simulink model "bh_4dof_LAGR_manipulator_CONTROL_DL_discrete"  (R2016b)
settings: Solver=ode15s  StartTime=0.0  StopTime=60  FixedStep=0.001  RelTol=1e-5  EnableMultiTasking=on
undefined symbols (not defined in the file or in its folder): b1_damp, b2_damp, b3_damp, b4_damp, g, Hz, L1x, L1y, L1z, L2x, L2y, L2z, L3x, L3y, L3z, mass1, mass2, mass3, mass4, Rturn, theta1_0, theta1_dot_0, theta2_0, theta2_dot_0, theta3_0, theta3_dot_0, theta4_0, theta4_dot_0, X, Y, Z
libraries: sm_lib x25, nesl_utility x17, simulink x9, discretizing x4, simulink_extras x2
(part 2 of 3)

== system bh_4dof_LAGR_manipulator_CONTROL_DL_discrete/CONTROL_LAW/CLAW_LINK2 ==
  note: Rise Settle
      | VEL LOOP 0.0056 0.01
      | POS LOOP 0.0274 0.05
  FFWD : Inport
  CMD_POS : Inport  Port=2
  MEAS_POS : Inport  Port=3
  MEAS_VEL : Inport  Port=4
  Constant : Constant
  Manual Switch : ManualSwitch  CurrentSetting=0
  PID Controller : simulink/Continuous/PID Controller  Controller=P  TimeDomain=Discrete-time  SampleTime=0.001  IntegratorMethod=Forward Euler  FilterMethod=Forward Euler  Form=Parallel  UseFilter=on  ControllerParametersSource=internal  P=64.6199485469639  I=1  D=0  N=100  InitialConditionSource=internal  InitialConditionForIntegrator=0  InitialConditionForFilter=0  ExternalReset=none  LimitOutput=off  UpperSaturationLimit=inf  LowerSaturationLimit=-inf  LinearizeAsGain=on  AntiWindupMode=none  Kb=1  TrackingMode=off  Kt=1  PParamMin=[]  PParamMax=[]  IParamMin=[]  IParamMax=[]  DParamMin=[]  DParamMax=[]  NParamMin=[]  NParamMax=[]  KbParamMin=[]  KbParamMax=[]  KtParamMin=[]  KtParamMax=[]  POutMin=[]  POutMax=[]  IOutMin=[]  IOutMax=[]  DOutMin=[]  DOutMax=[]  NOutMin=[]  NOutMax=[]  KbOutMin=[]  KbOutMax=[]  KtOutMin=[]  KtOutMax=[]  IntegratorOutMin=[]  IntegratorOutMax=[]  FilterOutMin=[]  FilterOutMax=[]  SumOutMin=[]  SumOutMax=[]  SumI1OutMin=[]  SumI1OutMax=[]  SumI2OutMin=[]  SumI2OutMax=[]  SumI3OutMin=[]  SumI3OutMax=[]  SumDOutMin=[]  SumDOutMax=[]  SaturationOutMin=[]  SaturationOutMax=[]  IntegratorContinuousStateAttributes=''  IntegratorStateMustResolveToSignalObject=off  IntegratorRTWStateStorageClass=Auto  FilterContinuousStateAttributes=''  FilterStateMustResolveToSignalObject=off  FilterRTWStateStorageClass=Auto  DifferentiatorICPrevScaledInput=0  DifferentiatorOutMin=[]  DifferentiatorOutMax=[]
      settings: AttributesFormatString=DT= %<SampleTime>
  PID Controller1 : simulink/Continuous/PID Controller  Controller=P  TimeDomain=Discrete-time  SampleTime=0.001  IntegratorMethod=Forward Euler  FilterMethod=Forward Euler  Form=Parallel  UseFilter=on  ControllerParametersSource=internal  P=12.0646813225273  I=10  D=0  N=100  InitialConditionSource=internal  InitialConditionForIntegrator=0  InitialConditionForFilter=0  ExternalReset=none  LimitOutput=off  UpperSaturationLimit=inf  LowerSaturationLimit=-inf  LinearizeAsGain=on  AntiWindupMode=none  Kb=1  TrackingMode=off  Kt=1  PParamMin=[]  PParamMax=[]  IParamMin=[]  IParamMax=[]  DParamMin=[]  DParamMax=[]  NParamMin=[]  NParamMax=[]  KbParamMin=[]  KbParamMax=[]  KtParamMin=[]  KtParamMax=[]  POutMin=[]  POutMax=[]  IOutMin=[]  IOutMax=[]  DOutMin=[]  DOutMax=[]  NOutMin=[]  NOutMax=[]  KbOutMin=[]  KbOutMax=[]  KtOutMin=[]  KtOutMax=[]  IntegratorOutMin=[]  IntegratorOutMax=[]  FilterOutMin=[]  FilterOutMax=[]  SumOutMin=[]  SumOutMax=[]  SumI1OutMin=[]  SumI1OutMax=[]  SumI2OutMin=[]  SumI2OutMax=[]  SumI3OutMin=[]  SumI3OutMax=[]  SumDOutMin=[]  SumDOutMax=[]  SaturationOutMin=[]  SaturationOutMax=[]  IntegratorContinuousStateAttributes=''  IntegratorStateMustResolveToSignalObject=off  IntegratorRTWStateStorageClass=Auto  FilterContinuousStateAttributes=''  FilterStateMustResolveToSignalObject=off  FilterRTWStateStorageClass=Auto  DifferentiatorICPrevScaledInput=0  DifferentiatorOutMin=[]  DifferentiatorOutMax=[]
      settings: AttributesFormatString=DT= %<SampleTime>
  Sum : Sum  Inputs=|+-
  Sum1 : Sum  Inputs=++|
  Sum2 : Sum  Inputs=+|-
  Transfer Fcn1 : discretizing/Discretized Transfer Fcn  Numerator=[100]  Denominator=[1 100]  AbsTol=auto  SampleTime=0.001  method=tustin  Wc=1
  Transfer Fcn4 : discretizing/Discretized Transfer Fcn  Commented=on  Numerator=[300]  Denominator=[1 300]  AbsTol=auto  SampleTime=0.001  method=tustin  Wc=1
  TQ : Outport
  wires:
  FFWD/1 -> Sum1/1
  Sum1/1 -> [T], TQ/1
  CMD_POS/1 -> Sum/1
  MEAS_VEL/1 -> Transfer Fcn1/1  "VEL"
  MEAS_POS/1 -> Sum/2  "POS"
  PID Controller/1 -> Manual Switch/2
  Sum2/1 -> PID Controller1/1
  Manual Switch/1 -> Sum2/1, [VZ]
  Constant/1 -> Manual Switch/1
  PID Controller1/1 -> Sum1/2
  Sum/1 -> PID Controller/1
  Transfer Fcn1/1 -> Sum2/2

== system bh_4dof_LAGR_manipulator_CONTROL_DL_discrete/CONTROL_LAW/CLAW_LINK3 ==
  note: Rise Settle
      | VEL LOOP 0.0056 0.01
      | POS LOOP 0.0274 0.05
  FFWD : Inport
  CMD_POS : Inport  Port=2
  MEAS_POS : Inport  Port=3
  MEAS_VEL : Inport  Port=4
  Constant : Constant
  Manual Switch : ManualSwitch  CurrentSetting=0
  PID Controller : simulink/Continuous/PID Controller  Controller=P  TimeDomain=Discrete-time  SampleTime=0.001  IntegratorMethod=Forward Euler  FilterMethod=Forward Euler  Form=Parallel  UseFilter=on  ControllerParametersSource=internal  P=15*4  I=1  D=0  N=100  InitialConditionSource=internal  InitialConditionForIntegrator=0  InitialConditionForFilter=0  ExternalReset=none  LimitOutput=off  UpperSaturationLimit=inf  LowerSaturationLimit=-inf  LinearizeAsGain=on  AntiWindupMode=none  Kb=1  TrackingMode=off  Kt=1  PParamMin=[]  PParamMax=[]  IParamMin=[]  IParamMax=[]  DParamMin=[]  DParamMax=[]  NParamMin=[]  NParamMax=[]  KbParamMin=[]  KbParamMax=[]  KtParamMin=[]  KtParamMax=[]  POutMin=[]  POutMax=[]  IOutMin=[]  IOutMax=[]  DOutMin=[]  DOutMax=[]  NOutMin=[]  NOutMax=[]  KbOutMin=[]  KbOutMax=[]  KtOutMin=[]  KtOutMax=[]  IntegratorOutMin=[]  IntegratorOutMax=[]  FilterOutMin=[]  FilterOutMax=[]  SumOutMin=[]  SumOutMax=[]  SumI1OutMin=[]  SumI1OutMax=[]  SumI2OutMin=[]  SumI2OutMax=[]  SumI3OutMin=[]  SumI3OutMax=[]  SumDOutMin=[]  SumDOutMax=[]  SaturationOutMin=[]  SaturationOutMax=[]  IntegratorContinuousStateAttributes=''  IntegratorStateMustResolveToSignalObject=off  IntegratorRTWStateStorageClass=Auto  FilterContinuousStateAttributes=''  FilterStateMustResolveToSignalObject=off  FilterRTWStateStorageClass=Auto  DifferentiatorICPrevScaledInput=0  DifferentiatorOutMin=[]  DifferentiatorOutMax=[]
      settings: AttributesFormatString=DT= %<SampleTime>
  PID Controller1 : simulink/Continuous/PID Controller  Controller=P  TimeDomain=Discrete-time  SampleTime=0.001  IntegratorMethod=Forward Euler  FilterMethod=Forward Euler  Form=Parallel  UseFilter=on  ControllerParametersSource=internal  P=0.422912648203834  I=10  D=0  N=100  InitialConditionSource=internal  InitialConditionForIntegrator=0  InitialConditionForFilter=0  ExternalReset=none  LimitOutput=off  UpperSaturationLimit=inf  LowerSaturationLimit=-inf  LinearizeAsGain=on  AntiWindupMode=none  Kb=1  TrackingMode=off  Kt=1  PParamMin=[]  PParamMax=[]  IParamMin=[]  IParamMax=[]  DParamMin=[]  DParamMax=[]  NParamMin=[]  NParamMax=[]  KbParamMin=[]  KbParamMax=[]  KtParamMin=[]  KtParamMax=[]  POutMin=[]  POutMax=[]  IOutMin=[]  IOutMax=[]  DOutMin=[]  DOutMax=[]  NOutMin=[]  NOutMax=[]  KbOutMin=[]  KbOutMax=[]  KtOutMin=[]  KtOutMax=[]  IntegratorOutMin=[]  IntegratorOutMax=[]  FilterOutMin=[]  FilterOutMax=[]  SumOutMin=[]  SumOutMax=[]  SumI1OutMin=[]  SumI1OutMax=[]  SumI2OutMin=[]  SumI2OutMax=[]  SumI3OutMin=[]  SumI3OutMax=[]  SumDOutMin=[]  SumDOutMax=[]  SaturationOutMin=[]  SaturationOutMax=[]  IntegratorContinuousStateAttributes=''  IntegratorStateMustResolveToSignalObject=off  IntegratorRTWStateStorageClass=Auto  FilterContinuousStateAttributes=''  FilterStateMustResolveToSignalObject=off  FilterRTWStateStorageClass=Auto  DifferentiatorICPrevScaledInput=0  DifferentiatorOutMin=[]  DifferentiatorOutMax=[]
      settings: AttributesFormatString=DT= %<SampleTime>
  Sum : Sum  Inputs=|+-
  Sum1 : Sum  Inputs=++|
  Sum2 : Sum  Inputs=+|-
  TQ : Outport
  wires:
  FFWD/1 -> Sum1/1
  Sum1/1 -> [T], TQ/1
  CMD_POS/1 -> Sum/1
  MEAS_VEL/1 -> Sum2/2  "VEL"
  MEAS_POS/1 -> Sum/2  "POS"
  Sum2/1 -> PID Controller1/1
  Manual Switch/1 -> Sum2/1, [VZ]
  Constant/1 -> Manual Switch/1
  Sum/1 -> PID Controller/1
  PID Controller1/1 -> Sum1/2
  PID Controller/1 -> Manual Switch/2

== system bh_4dof_LAGR_manipulator_CONTROL_DL_discrete/CONTROL_LAW/CLAW_TURN ==
  note: Settle
      | VEL LOOP 0.01
      | POS LOOP 0.05
  FFWD : Inport
  CMD_POS : Inport  Port=2
  MEAS_POS : Inport  Port=3
  MEAS_VEL : Inport  Port=4
  Constant : Constant
  Manual Switch : ManualSwitch  CurrentSetting=0
  PID Controller : simulink/Continuous/PID Controller  Controller=P  TimeDomain=Discrete-time  SampleTime=0.001  IntegratorMethod=Forward Euler  FilterMethod=Forward Euler  Form=Parallel  UseFilter=on  ControllerParametersSource=internal  P=63.9206057044755  I=1  D=0  N=100  InitialConditionSource=internal  InitialConditionForIntegrator=0  InitialConditionForFilter=0  ExternalReset=none  LimitOutput=off  UpperSaturationLimit=inf  LowerSaturationLimit=-inf  LinearizeAsGain=on  AntiWindupMode=none  Kb=1  TrackingMode=off  Kt=1  PParamMin=[]  PParamMax=[]  IParamMin=[]  IParamMax=[]  DParamMin=[]  DParamMax=[]  NParamMin=[]  NParamMax=[]  KbParamMin=[]  KbParamMax=[]  KtParamMin=[]  KtParamMax=[]  POutMin=[]  POutMax=[]  IOutMin=[]  IOutMax=[]  DOutMin=[]  DOutMax=[]  NOutMin=[]  NOutMax=[]  KbOutMin=[]  KbOutMax=[]  KtOutMin=[]  KtOutMax=[]  IntegratorOutMin=[]  IntegratorOutMax=[]  FilterOutMin=[]  FilterOutMax=[]  SumOutMin=[]  SumOutMax=[]  SumI1OutMin=[]  SumI1OutMax=[]  SumI2OutMin=[]  SumI2OutMax=[]  SumI3OutMin=[]  SumI3OutMax=[]  SumDOutMin=[]  SumDOutMax=[]  SaturationOutMin=[]  SaturationOutMax=[]  IntegratorContinuousStateAttributes=''  IntegratorStateMustResolveToSignalObject=off  IntegratorRTWStateStorageClass=Auto  FilterContinuousStateAttributes=''  FilterStateMustResolveToSignalObject=off  FilterRTWStateStorageClass=Auto  DifferentiatorICPrevScaledInput=0  DifferentiatorOutMin=[]  DifferentiatorOutMax=[]
      settings: AttributesFormatString=DT= %<SampleTime>
  PID Controller1 : simulink/Continuous/PID Controller  Controller=P  TimeDomain=Discrete-time  SampleTime=0.001  IntegratorMethod=Forward Euler  FilterMethod=Forward Euler  Form=Parallel  UseFilter=on  ControllerParametersSource=internal  P=91.9060817614885  I=10  D=0  N=100  InitialConditionSource=internal  InitialConditionForIntegrator=0  InitialConditionForFilter=0  ExternalReset=none  LimitOutput=off  UpperSaturationLimit=inf  LowerSaturationLimit=-inf  LinearizeAsGain=on  AntiWindupMode=none  Kb=1  TrackingMode=off  Kt=1  PParamMin=[]  PParamMax=[]  IParamMin=[]  IParamMax=[]  DParamMin=[]  DParamMax=[]  NParamMin=[]  NParamMax=[]  KbParamMin=[]  KbParamMax=[]  KtParamMin=[]  KtParamMax=[]  POutMin=[]  POutMax=[]  IOutMin=[]  IOutMax=[]  DOutMin=[]  DOutMax=[]  NOutMin=[]  NOutMax=[]  KbOutMin=[]  KbOutMax=[]  KtOutMin=[]  KtOutMax=[]  IntegratorOutMin=[]  IntegratorOutMax=[]  FilterOutMin=[]  FilterOutMax=[]  SumOutMin=[]  SumOutMax=[]  SumI1OutMin=[]  SumI1OutMax=[]  SumI2OutMin=[]  SumI2OutMax=[]  SumI3OutMin=[]  SumI3OutMax=[]  SumDOutMin=[]  SumDOutMax=[]  SaturationOutMin=[]  SaturationOutMax=[]  IntegratorContinuousStateAttributes=''  IntegratorStateMustResolveToSignalObject=off  IntegratorRTWStateStorageClass=Auto  FilterContinuousStateAttributes=''  FilterStateMustResolveToSignalObject=off  FilterRTWStateStorageClass=Auto  DifferentiatorICPrevScaledInput=0  DifferentiatorOutMin=[]  DifferentiatorOutMax=[]
      settings: AttributesFormatString=DT= %<SampleTime>
  Sum : Sum  Inputs=|+-
  Sum1 : Sum  Inputs=++|
  Sum2 : Sum  Inputs=+|-
  TQ : Outport
  wires:
  FFWD/1 -> Sum1/1
  Sum1/1 -> [T], TQ/1
  CMD_POS/1 -> Sum/1
  MEAS_VEL/1 -> Sum2/2  "VEL"
  MEAS_POS/1 -> Sum/2  "POS"
  PID Controller/1 -> Manual Switch/2
  Sum2/1 -> PID Controller1/1
  Manual Switch/1 -> Sum2/1, [VZ]
  Constant/1 -> Manual Switch/1
  PID Controller1/1 -> Sum1/2
  Sum/1 -> PID Controller/1

== system bh_4dof_LAGR_manipulator_CONTROL_DL_discrete/CONTROL_LAW/Subsystem ==
  In1 : Inport
  Bus Assignment : BusAssignment  AssignedSignals=MEAS_BUS.TH_VEL
  Bus Selector4 : BusSelector  OutputSignals=MEAS_BUS.TH_VEL
  Mux : Mux
  Reshape : Reshape  OutputDimensionality=Column vector (2-D)
  Selector : Selector  InputPortWidth=4  IndexOptions=Index vector (dialog)  Indices=1  OutputSizes=1
  Selector1 : Selector  InputPortWidth=4  IndexOptions=Index vector (dialog)  Indices=2  OutputSizes=1
  Selector2 : Selector  InputPortWidth=4  IndexOptions=Index vector (dialog)  Indices=3  OutputSizes=1
  Selector3 : Selector  InputPortWidth=4  IndexOptions=Index vector (dialog)  Indices=4  OutputSizes=1
  Transfer Fcn{1..4} (4 alike) : TransferFcn  Numerator=[300]  Denominator=[1 300]
  Zero-Order Hold{1..4} (4 alike) : ZeroOrderHold  SampleTime=0.001
      settings: AttributesFormatString=DT =%<SampleTime>
  Out1 : Outport
  wires:
  In1/1 -> Bus Assignment/1, Bus Selector4/1
  Bus Selector4/1 -> Selector3/1, Selector2/1, Selector1/1, Selector/1  "<TH_VEL>"
  Transfer Fcn4/1 -> Mux/4
  Transfer Fcn1/1 -> Mux/3
  Transfer Fcn2/1 -> Mux/2
  Transfer Fcn3/1 -> Mux/1
  Mux/1 -> Reshape/1
  Bus Assignment/1 -> Out1/1
  Reshape/1 -> Bus Assignment/2
  Selector/1 -> Zero-Order Hold1/1
  Zero-Order Hold1/1 -> Transfer Fcn3/1
  Selector3/1 -> Zero-Order Hold4/1
  Selector2/1 -> Zero-Order Hold3/1
  Selector1/1 -> Zero-Order Hold2/1
  Zero-Order Hold2/1 -> Transfer Fcn2/1
  Zero-Order Hold3/1 -> Transfer Fcn1/1
  Zero-Order Hold4/1 -> Transfer Fcn4/1

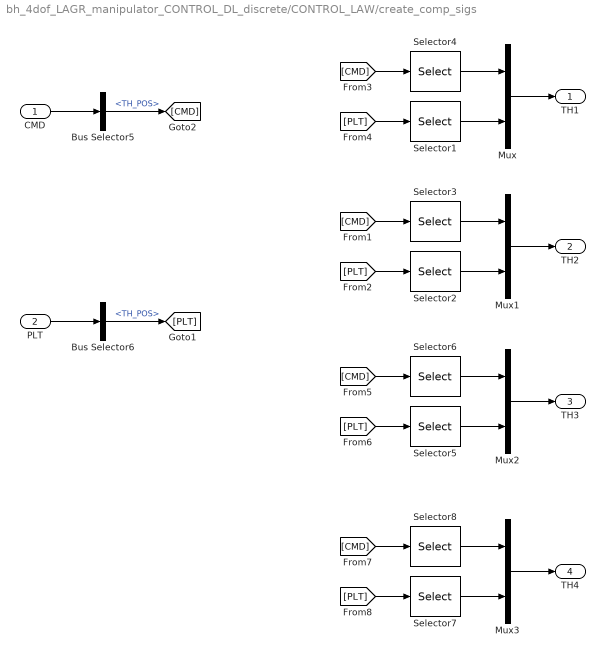
== system bh_4dof_LAGR_manipulator_CONTROL_DL_discrete/CONTROL_LAW/create_comp_sigs ==
  CMD : Inport
  PLT : Inport  Port=2
  Bus Selector5 : BusSelector  OutputSignals=TH_POS
  Bus Selector6 : BusSelector  OutputSignals=MEAS_BUS.TH_POS
  Mux{,1..3} (4 alike) : Mux  Inputs=2
  Selector1 : Selector  InputPortWidth=4  IndexOptions=Index vector (dialog)  Indices=1  OutputSizes=1
  Selector2 : Selector  InputPortWidth=4  IndexOptions=Index vector (dialog)  Indices=2  OutputSizes=1
  Selector3 : Selector  InputPortWidth=4  IndexOptions=Index vector (dialog)  Indices=2  OutputSizes=1
  Selector4 : Selector  InputPortWidth=4  IndexOptions=Index vector (dialog)  Indices=1  OutputSizes=1
  Selector5 : Selector  InputPortWidth=4  IndexOptions=Index vector (dialog)  Indices=3  OutputSizes=1
  Selector6 : Selector  InputPortWidth=4  IndexOptions=Index vector (dialog)  Indices=3  OutputSizes=1
  Selector7 : Selector  InputPortWidth=4  IndexOptions=Index vector (dialog)  Indices=4  OutputSizes=1
  Selector8 : Selector  InputPortWidth=4  IndexOptions=Index vector (dialog)  Indices=4  OutputSizes=1
  TH1 : Outport
  TH2 : Outport  Port=2
  TH3 : Outport  Port=3
  TH4 : Outport  Port=4
  wires:
  PLT/1 -> Bus Selector6/1
  Bus Selector6/1 -> [PLT]  "<TH_POS>"
  CMD/1 -> Bus Selector5/1
  Bus Selector5/1 -> [CMD]  "<TH_POS>"
  [CMD] -> Selector4/1
  Selector1/1 -> Mux/2
  Selector4/1 -> Mux/1
  [PLT] -> Selector1/1
  Mux/1 -> TH1/1
  [CMD] -> Selector3/1
  Selector2/1 -> Mux1/2
  Selector3/1 -> Mux1/1
  [PLT] -> Selector2/1
  Mux1/1 -> TH2/1
  [CMD] -> Selector6/1
  Selector5/1 -> Mux2/2
  Selector6/1 -> Mux2/1
  [PLT] -> Selector5/1
  Mux2/1 -> TH3/1
  [CMD] -> Selector8/1
  Selector7/1 -> Mux3/2
  Selector8/1 -> Mux3/1
  [PLT] -> Selector7/1
  Mux3/1 -> TH4/1

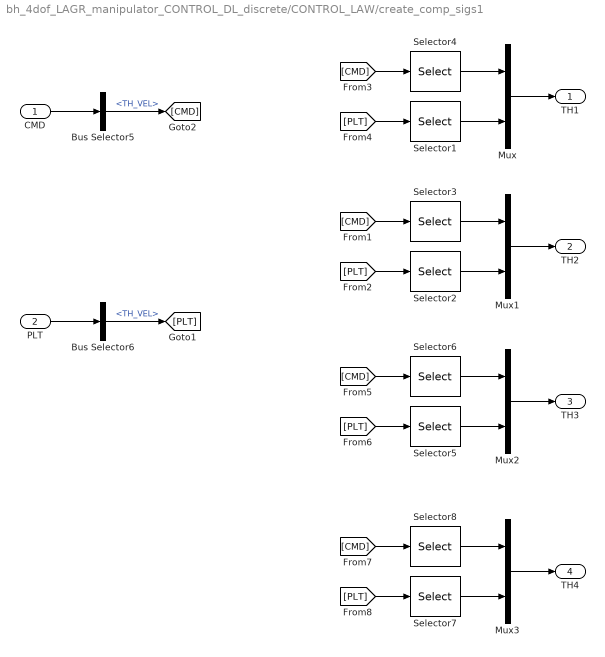
== system bh_4dof_LAGR_manipulator_CONTROL_DL_discrete/CONTROL_LAW/create_comp_sigs1 ==
  CMD : Inport
  PLT : Inport  Port=2
  Bus Selector5 : BusSelector  OutputSignals=TH_VEL
  Bus Selector6 : BusSelector  OutputSignals=MEAS_BUS.TH_VEL
  Mux{,1..3} (4 alike) : Mux  Inputs=2
  Selector1 : Selector  InputPortWidth=4  IndexOptions=Index vector (dialog)  Indices=1  OutputSizes=1
  Selector2 : Selector  InputPortWidth=4  IndexOptions=Index vector (dialog)  Indices=2  OutputSizes=1
  Selector3 : Selector  InputPortWidth=4  IndexOptions=Index vector (dialog)  Indices=2  OutputSizes=1
  Selector4 : Selector  InputPortWidth=4  IndexOptions=Index vector (dialog)  Indices=1  OutputSizes=1
  Selector5 : Selector  InputPortWidth=4  IndexOptions=Index vector (dialog)  Indices=3  OutputSizes=1
  Selector6 : Selector  InputPortWidth=4  IndexOptions=Index vector (dialog)  Indices=3  OutputSizes=1
  Selector7 : Selector  InputPortWidth=4  IndexOptions=Index vector (dialog)  Indices=4  OutputSizes=1
  Selector8 : Selector  InputPortWidth=4  IndexOptions=Index vector (dialog)  Indices=4  OutputSizes=1
  TH1 : Outport
  TH2 : Outport  Port=2
  TH3 : Outport  Port=3
  TH4 : Outport  Port=4
  wires:
  PLT/1 -> Bus Selector6/1
  Bus Selector6/1 -> [PLT]  "<TH_VEL>"
  CMD/1 -> Bus Selector5/1
  Bus Selector5/1 -> [CMD]  "<TH_VEL>"
  [CMD] -> Selector4/1
  Selector1/1 -> Mux/2
  Selector4/1 -> Mux/1
  [PLT] -> Selector1/1
  Mux/1 -> TH1/1
  [CMD] -> Selector3/1
  Selector2/1 -> Mux1/2
  Selector3/1 -> Mux1/1
  [PLT] -> Selector2/1
  Mux1/1 -> TH2/1
  [CMD] -> Selector6/1
  Selector5/1 -> Mux2/2
  Selector6/1 -> Mux2/1
  [PLT] -> Selector5/1
  Mux2/1 -> TH3/1
  [CMD] -> Selector8/1
  Selector7/1 -> Mux3/2
  Selector8/1 -> Mux3/1
  [PLT] -> Selector7/1
  Mux3/1 -> TH4/1

== system bh_4dof_LAGR_manipulator_CONTROL_DL_discrete/Create_PLANT_BUS/CALC_BUS ==
  MODEL_BUS : Inport
  Bus Creator : BusCreator  Inputs=14
  Bus Selector : BusSelector  OutputSignals=TH1,TH2,TH3,TH4
  Bus Selector1 : BusSelector  OutputSignals=TH1,TH2,TH3
  Constant1 : Constant  Value=L2y
  Constant17 : Constant  Value=L2y
  Constant18 : Constant  Value=L1y
  Constant19 : Constant  Value=L3y
  Constant2 : Constant  Value=L1y
  Constant3 : Constant  Value=L3y
  THE_A_EFF_and_O_and_G : MATLAB Function  TreatAsAtomicUnit=on
  THE_W_EFF_and_O_and_G : MATLAB Function  TreatAsAtomicUnit=on
  CALC_POS : Outport
  wires:
  Bus Selector/1 -> THE_W_EFF_and_O_and_G/4(theta1)  "<TH1>"
  Bus Selector/2 -> THE_W_EFF_and_O_and_G/5(theta2)  "<TH2>"
  Bus Selector/3 -> THE_W_EFF_and_O_and_G/6(theta3)  "<TH3>"
  Bus Selector/4 -> THE_W_EFF_and_O_and_G/7(theta4)  "<TH4>"
  Bus Creator/1 -> CALC_POS/1
  Constant18/1 -> THE_W_EFF_and_O_and_G/1(L1Y_s)
  Constant17/1 -> THE_W_EFF_and_O_and_G/2(L2Y_s)
  Constant19/1 -> THE_W_EFF_and_O_and_G/3(L3Y_s)
  THE_W_EFF_and_O_and_G/4(WF_pos_O3) -> Bus Creator/4  "WF_pos_O3"
  THE_W_EFF_and_O_and_G/6(WF_pos_G2) -> Bus Creator/6  "WF_pos_G2"
  THE_W_EFF_and_O_and_G/3(WF_pos_O2) -> Bus Creator/3  "WF_pos_O2"
  THE_W_EFF_and_O_and_G/7(WF_pos_G3) -> Bus Creator/7  "WF_pos_G3"
  THE_W_EFF_and_O_and_G/1(WF_pos_eff) -> Bus Creator/1  "WF_pos_EFF"
  THE_W_EFF_and_O_and_G/5(WF_pos_G1) -> Bus Creator/5  "WF_pos_G1"
  THE_W_EFF_and_O_and_G/2(WF_pos_O1) -> Bus Creator/2  "WF_pos_O1"
  MODEL_BUS/1 -> Bus Selector1/1, Bus Selector/1
  Bus Selector1/1 -> THE_A_EFF_and_O_and_G/4(theta1)  "<TH1>"
  Bus Selector1/2 -> THE_A_EFF_and_O_and_G/5(theta2)  "<TH2>"
  Bus Selector1/3 -> THE_A_EFF_and_O_and_G/6(theta3)  "<TH3>"
  Constant2/1 -> THE_A_EFF_and_O_and_G/1(L1Y_s)
  Constant1/1 -> THE_A_EFF_and_O_and_G/2(L2Y_s)
  Constant3/1 -> THE_A_EFF_and_O_and_G/3(L3Y_s)
  THE_A_EFF_and_O_and_G/7(AF_pos_G3) -> Bus Creator/14  "AF_pos_G3"
  THE_A_EFF_and_O_and_G/6(AF_pos_G2) -> Bus Creator/13  "AF_pos_G2"
  THE_A_EFF_and_O_and_G/5(AF_pos_G1) -> Bus Creator/12  "AF_pos_G1"
  THE_A_EFF_and_O_and_G/4(AF_pos_O3) -> Bus Creator/11  "AF_pos_O3"
  THE_A_EFF_and_O_and_G/3(AF_pos_O2) -> Bus Creator/10  "AF_pos_O2"
  THE_A_EFF_and_O_and_G/2(AF_pos_O1) -> Bus Creator/9  "AF_pos_O1"
  THE_A_EFF_and_O_and_G/1(AF_pos_eff) -> Bus Creator/8  "AF_pos_EFF"

== system bh_4dof_LAGR_manipulator_CONTROL_DL_discrete/Create_PLANT_BUS/MEAS ==
  MODEL_BUS : Inport
  Bus Creator : BusCreator  Inputs=3
  Bus Selector : BusSelector  OutputSignals=TH1,TH2,TH3,TH4
  Bus Selector1 : BusSelector  OutputSignals=TH1_D,TH2_D,TH3_D,TH4_D
  Bus Selector2 : BusSelector  OutputSignals=TH1_DD,TH2_DD,TH3_DD,TH4_DD
  Mux : Mux
  Mux1 : Mux
  Mux2 : Mux
  Reshape : Reshape  OutputDimensionality=Column vector (2-D)
  Reshape1 : Reshape  OutputDimensionality=Column vector (2-D)
  Reshape2 : Reshape  OutputDimensionality=Column vector (2-D)
  MEAS : Outport
  wires:
  MODEL_BUS/1 -> Bus Selector/1, Bus Selector2/1, Bus Selector1/1
  Bus Selector/1 -> Mux/1  "<TH1>"
  Bus Selector/2 -> Mux/2  "<TH2>"
  Bus Selector/3 -> Mux/3  "<TH3>"
  Bus Selector/4 -> Mux/4  "<TH4>"
  Bus Selector1/1 -> Mux1/1  "<TH1_D>"
  Bus Selector1/2 -> Mux1/2  "<TH2_D>"
  Bus Selector1/3 -> Mux1/3  "<TH3_D>"
  Bus Selector1/4 -> Mux1/4  "<TH4_D>"
  Bus Selector2/1 -> Mux2/1  "<TH1_DD>"
  Bus Selector2/2 -> Mux2/2  "<TH2_DD>"
  Bus Selector2/3 -> Mux2/3  "<TH3_DD>"
  Bus Selector2/4 -> Mux2/4  "<TH4_DD>"
  Mux/1 -> Reshape/1  "TH_POS"
  Mux1/1 -> Reshape1/1  "TH_VEL"
  Mux2/1 -> Reshape2/1  "TH_ACC"
  Reshape/1 -> Bus Creator/1  "TH_POS"
  Reshape1/1 -> Bus Creator/2  "TH_VEL"
  Reshape2/1 -> Bus Creator/3  "TH_ACC"
  Bus Creator/1 -> MEAS/1

== system bh_4dof_LAGR_manipulator_CONTROL_DL_discrete/Create_PLANT_BUS/Subsystem ==
  MODEL : Inport
  MEAS : Inport  Port=2
  CALC_POS : Inport  Port=3
  CALC_GRAV_TQ : Inport  Port=4
  Bus Creator : BusCreator  Inputs=4
  PLANT_B : Outport
  wires:
  MODEL/1 -> Bus Creator/1  "MODEL_BUS"
  MEAS/1 -> Bus Creator/2  "MEAS_BUS"
  CALC_POS/1 -> Bus Creator/3  "CALC_POS_BUS"
  Bus Creator/1 -> PLANT_B/1
  CALC_GRAV_TQ/1 -> Bus Creator/4  "CALC_GRAV_TQ_BUS"

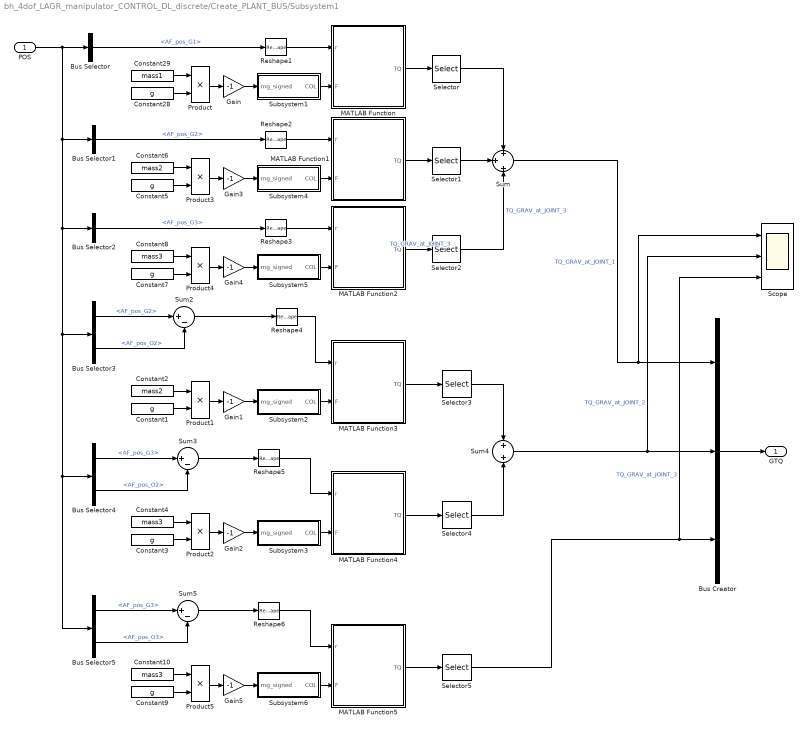
== system bh_4dof_LAGR_manipulator_CONTROL_DL_discrete/Create_PLANT_BUS/Subsystem1 ==
  POS : Inport
  Bus Creator : BusCreator  Inputs=3
  Bus Selector : BusSelector  OutputSignals=AF_pos_G1
  Bus Selector1 : BusSelector  OutputSignals=AF_pos_G2
  Bus Selector2 : BusSelector  OutputSignals=AF_pos_G3
  Bus Selector3 : BusSelector  OutputSignals=AF_pos_G2,AF_pos_O2
  Bus Selector4 : BusSelector  OutputSignals=AF_pos_G3,AF_pos_O2
  Bus Selector5 : BusSelector  OutputSignals=AF_pos_G3,AF_pos_O3
  Constant{1,3,5,7,9,28} (6 alike) : Constant  Value=g
  Constant10 : Constant  Value=mass3
  Constant2 : Constant  Value=mass2
  Constant29 : Constant  Value=mass1
  Constant4 : Constant  Value=mass3
  Constant6 : Constant  Value=mass2
  Constant8 : Constant  Value=mass3
  Gain{,1..5} (6 alike) : Gain  Gain=-1
  MATLAB Function : MATLAB Function  TreatAsAtomicUnit=on
  MATLAB Function1 : MATLAB Function  TreatAsAtomicUnit=on
  MATLAB Function2 : MATLAB Function  TreatAsAtomicUnit=on
  MATLAB Function3 : MATLAB Function  TreatAsAtomicUnit=on
  MATLAB Function4 : MATLAB Function  TreatAsAtomicUnit=on
  MATLAB Function5 : MATLAB Function  TreatAsAtomicUnit=on
  Product{,1..5} (6 alike) : Product
  Reshape{1..6} (6 alike) : Reshape  OutputDimensionality=Column vector (2-D)
  Scope : Scope  NumInputPorts=3
  Selector{,1..5} (6 alike) : Selector  InputPortWidth=3  IndexOptions=Index vector (dialog)  Indices=1  OutputSizes=1
  Subsystem1 : Subsystem
  Subsystem2 : Subsystem
  Subsystem3 : Subsystem
  Subsystem4 : Subsystem
  Subsystem5 : Subsystem
  Subsystem6 : Subsystem
  Sum : Sum  Inputs=+|+|+
  Sum2 : Sum  Inputs=|+-
  Sum3 : Sum  Inputs=|+-
  Sum4 : Sum  Inputs=+|+
  Sum5 : Sum  Inputs=|+-
  GTQ : Outport
  wires:
  Bus Selector/1 -> Reshape1/1  "<AF_pos_G1>"
  Constant29/1 -> Product/1
  Constant28/1 -> Product/2
  Product/1 -> Gain/1
  Gain/1 -> Subsystem1/1(mg_signed)
  Subsystem1/1(COL) -> MATLAB Function/2(F)
  Reshape1/1 -> MATLAB Function/1(r)
  Bus Selector1/1 -> Reshape2/1  "<AF_pos_G2>"
  Constant6/1 -> Product3/1
  Constant5/1 -> Product3/2
  Product3/1 -> Gain3/1
  Gain3/1 -> Subsystem4/1(mg_signed)
  Subsystem4/1(COL) -> MATLAB Function1/2(F)
  Reshape2/1 -> MATLAB Function1/1(r)
  Bus Selector2/1 -> Reshape3/1  "<AF_pos_G3>"
  Constant8/1 -> Product4/1
  Constant7/1 -> Product4/2
  Product4/1 -> Gain4/1
  Gain4/1 -> Subsystem5/1(mg_signed)
  Subsystem5/1(COL) -> MATLAB Function2/2(F)
  Reshape3/1 -> MATLAB Function2/1(r)
  MATLAB Function/1(TQ) -> Selector/1
  MATLAB Function2/1(TQ) -> Selector2/1  "TQ_GRAV_at_JOINT_3"
  MATLAB Function1/1(TQ) -> Selector1/1
  Bus Creator/1 -> GTQ/1
  Selector/1 -> Sum/1
  Selector1/1 -> Sum/2
  Selector2/1 -> Sum/3  "TQ_GRAV_at_JOINT_3"
  Bus Selector3/1 -> Sum2/1  "<AF_pos_G2>"
  Constant2/1 -> Product1/1
  Constant1/1 -> Product1/2
  Product1/1 -> Gain1/1
  Gain1/1 -> Subsystem2/1(mg_signed)
  Subsystem2/1(COL) -> MATLAB Function3/2(F)
  Reshape4/1 -> MATLAB Function3/1(r)
  Bus Selector4/1 -> Sum3/1  "<AF_pos_G3>"
  Constant4/1 -> Product2/1
  Constant3/1 -> Product2/2
  Product2/1 -> Gain2/1
  Gain2/1 -> Subsystem3/1(mg_signed)
  Subsystem3/1(COL) -> MATLAB Function4/2(F)
  Reshape5/1 -> MATLAB Function4/1(r)
  Sum2/1 -> Reshape4/1
  Bus Selector3/2 -> Sum2/2  "<AF_pos_O2>"
  Bus Selector4/2 -> Sum3/2  "<AF_pos_O2>"
  Sum3/1 -> Reshape5/1
  MATLAB Function3/1(TQ) -> Selector3/1
  MATLAB Function4/1(TQ) -> Selector4/1
  Selector3/1 -> Sum4/1
  Selector4/1 -> Sum4/2
  POS/1 -> Bus Selector5/1, Bus Selector4/1, Bus Selector3/1, Bus Selector2/1, Bus Selector1/1, Bus Selector/1
  Bus Selector5/1 -> Sum5/1  "<AF_pos_G3>"
  Constant10/1 -> Product5/1
  Constant9/1 -> Product5/2
  Product5/1 -> Gain5/1
  Gain5/1 -> Subsystem6/1(mg_signed)
  Subsystem6/1(COL) -> MATLAB Function5/2(F)
  Reshape6/1 -> MATLAB Function5/1(r)
  Bus Selector5/2 -> Sum5/2  "<AF_pos_O3>"
  Sum5/1 -> Reshape6/1
  MATLAB Function5/1(TQ) -> Selector5/1
  Sum4/1 -> Scope/2, Bus Creator/2  "TQ_GRAV_at_JOINT_2"
  Sum/1 -> Scope/1, Bus Creator/1  "TQ_GRAV_at_JOINT_1"
  Selector5/1 -> Scope/3, Bus Creator/3  "TQ_GRAV_at_JOINT_3"

== system bh_4dof_LAGR_manipulator_CONTROL_DL_discrete/Create_PLANT_BUS1/CALC_BUS ==
  MODEL_BUS : Inport
  Bus Creator : BusCreator  Inputs=14
  Bus Selector : BusSelector  OutputSignals=TH1,TH2,TH3,TH4
  Bus Selector1 : BusSelector  OutputSignals=TH1,TH2,TH3
  Constant1 : Constant  Value=L2y
  Constant17 : Constant  Value=L2y
  Constant18 : Constant  Value=L1y
  Constant19 : Constant  Value=L3y
  Constant2 : Constant  Value=L1y
  Constant3 : Constant  Value=L3y
  THE_A_EFF_and_O_and_G : MATLAB Function  TreatAsAtomicUnit=on
  THE_W_EFF_and_O_and_G : MATLAB Function  TreatAsAtomicUnit=on
  CALC_POS : Outport
  wires:
  Bus Selector/1 -> THE_W_EFF_and_O_and_G/4(theta1)  "<TH1>"
  Bus Selector/2 -> THE_W_EFF_and_O_and_G/5(theta2)  "<TH2>"
  Bus Selector/3 -> THE_W_EFF_and_O_and_G/6(theta3)  "<TH3>"
  Bus Selector/4 -> THE_W_EFF_and_O_and_G/7(theta4)  "<TH4>"
  Bus Creator/1 -> CALC_POS/1
  Constant18/1 -> THE_W_EFF_and_O_and_G/1(L1Y_s)
  Constant17/1 -> THE_W_EFF_and_O_and_G/2(L2Y_s)
  Constant19/1 -> THE_W_EFF_and_O_and_G/3(L3Y_s)
  THE_W_EFF_and_O_and_G/4(WF_pos_O3) -> Bus Creator/4  "WF_pos_O3"
  THE_W_EFF_and_O_and_G/6(WF_pos_G2) -> Bus Creator/6  "WF_pos_G2"
  THE_W_EFF_and_O_and_G/3(WF_pos_O2) -> Bus Creator/3  "WF_pos_O2"
  THE_W_EFF_and_O_and_G/7(WF_pos_G3) -> Bus Creator/7  "WF_pos_G3"
  THE_W_EFF_and_O_and_G/1(WF_pos_eff) -> Bus Creator/1  "WF_pos_EFF"
  THE_W_EFF_and_O_and_G/5(WF_pos_G1) -> Bus Creator/5  "WF_pos_G1"
  THE_W_EFF_and_O_and_G/2(WF_pos_O1) -> Bus Creator/2  "WF_pos_O1"
  MODEL_BUS/1 -> Bus Selector1/1, Bus Selector/1
  Bus Selector1/1 -> THE_A_EFF_and_O_and_G/4(theta1)  "<TH1>"
  Bus Selector1/2 -> THE_A_EFF_and_O_and_G/5(theta2)  "<TH2>"
  Bus Selector1/3 -> THE_A_EFF_and_O_and_G/6(theta3)  "<TH3>"
  Constant2/1 -> THE_A_EFF_and_O_and_G/1(L1Y_s)
  Constant1/1 -> THE_A_EFF_and_O_and_G/2(L2Y_s)
  Constant3/1 -> THE_A_EFF_and_O_and_G/3(L3Y_s)
  THE_A_EFF_and_O_and_G/7(AF_pos_G3) -> Bus Creator/14  "AF_pos_G3"
  THE_A_EFF_and_O_and_G/6(AF_pos_G2) -> Bus Creator/13  "AF_pos_G2"
  THE_A_EFF_and_O_and_G/5(AF_pos_G1) -> Bus Creator/12  "AF_pos_G1"
  THE_A_EFF_and_O_and_G/4(AF_pos_O3) -> Bus Creator/11  "AF_pos_O3"
  THE_A_EFF_and_O_and_G/3(AF_pos_O2) -> Bus Creator/10  "AF_pos_O2"
  THE_A_EFF_and_O_and_G/2(AF_pos_O1) -> Bus Creator/9  "AF_pos_O1"
  THE_A_EFF_and_O_and_G/1(AF_pos_eff) -> Bus Creator/8  "AF_pos_EFF"

== system bh_4dof_LAGR_manipulator_CONTROL_DL_discrete/Create_PLANT_BUS1/MEAS ==
  MODEL_BUS : Inport
  Bus Creator : BusCreator  Inputs=3
  Bus Selector : BusSelector  OutputSignals=TH1,TH2,TH3,TH4
  Bus Selector1 : BusSelector  OutputSignals=TH1_D,TH2_D,TH3_D,TH4_D
  Bus Selector2 : BusSelector  OutputSignals=TH1_DD,TH2_DD,TH3_DD,TH4_DD
  Mux : Mux
  Mux1 : Mux
  Mux2 : Mux
  Reshape : Reshape  OutputDimensionality=Column vector (2-D)
  Reshape1 : Reshape  OutputDimensionality=Column vector (2-D)
  Reshape2 : Reshape  OutputDimensionality=Column vector (2-D)
  MEAS : Outport
  wires:
  MODEL_BUS/1 -> Bus Selector/1, Bus Selector2/1, Bus Selector1/1
  Bus Selector/1 -> Mux/1  "<TH1>"
  Bus Selector/2 -> Mux/2  "<TH2>"
  Bus Selector/3 -> Mux/3  "<TH3>"
  Bus Selector/4 -> Mux/4  "<TH4>"
  Bus Selector1/1 -> Mux1/1  "<TH1_D>"
  Bus Selector1/2 -> Mux1/2  "<TH2_D>"
  Bus Selector1/3 -> Mux1/3  "<TH3_D>"
  Bus Selector1/4 -> Mux1/4  "<TH4_D>"
  Bus Selector2/1 -> Mux2/1  "<TH1_DD>"
  Bus Selector2/2 -> Mux2/2  "<TH2_DD>"
  Bus Selector2/3 -> Mux2/3  "<TH3_DD>"
  Bus Selector2/4 -> Mux2/4  "<TH4_DD>"
  Mux/1 -> Reshape/1  "TH_POS"
  Mux1/1 -> Reshape1/1  "TH_VEL"
  Mux2/1 -> Reshape2/1  "TH_ACC"
  Reshape/1 -> Bus Creator/1  "TH_POS"
  Reshape1/1 -> Bus Creator/2  "TH_VEL"
  Reshape2/1 -> Bus Creator/3  "TH_ACC"
  Bus Creator/1 -> MEAS/1

== system bh_4dof_LAGR_manipulator_CONTROL_DL_discrete/Create_PLANT_BUS1/Subsystem ==
  MODEL : Inport
  MEAS : Inport  Port=2
  CALC_POS : Inport  Port=3
  CALC_GRAV_TQ : Inport  Port=4
  Bus Creator : BusCreator  Inputs=4
  PLANT_B : Outport
  wires:
  MODEL/1 -> Bus Creator/1  "MODEL_BUS"
  MEAS/1 -> Bus Creator/2  "MEAS_BUS"
  CALC_POS/1 -> Bus Creator/3  "CALC_POS_BUS"
  Bus Creator/1 -> PLANT_B/1
  CALC_GRAV_TQ/1 -> Bus Creator/4  "CALC_GRAV_TQ_BUS"

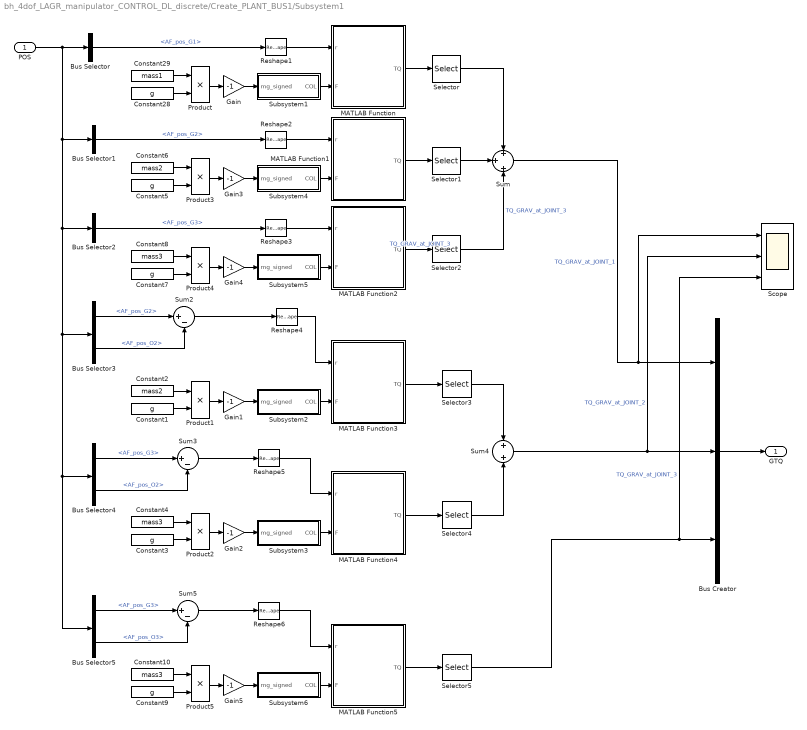
== system bh_4dof_LAGR_manipulator_CONTROL_DL_discrete/Create_PLANT_BUS1/Subsystem1 ==
  POS : Inport
  Bus Creator : BusCreator  Inputs=3
  Bus Selector : BusSelector  OutputSignals=AF_pos_G1
  Bus Selector1 : BusSelector  OutputSignals=AF_pos_G2
  Bus Selector2 : BusSelector  OutputSignals=AF_pos_G3
  Bus Selector3 : BusSelector  OutputSignals=AF_pos_G2,AF_pos_O2
  Bus Selector4 : BusSelector  OutputSignals=AF_pos_G3,AF_pos_O2
  Bus Selector5 : BusSelector  OutputSignals=AF_pos_G3,AF_pos_O3
  Constant{1,3,5,7,9,28} (6 alike) : Constant  Value=g
  Constant10 : Constant  Value=mass3
  Constant2 : Constant  Value=mass2
  Constant29 : Constant  Value=mass1
  Constant4 : Constant  Value=mass3
  Constant6 : Constant  Value=mass2
  Constant8 : Constant  Value=mass3
  Gain{,1..5} (6 alike) : Gain  Gain=-1
  MATLAB Function : MATLAB Function  TreatAsAtomicUnit=on
  MATLAB Function1 : MATLAB Function  TreatAsAtomicUnit=on
  MATLAB Function2 : MATLAB Function  TreatAsAtomicUnit=on
  MATLAB Function3 : MATLAB Function  TreatAsAtomicUnit=on
  MATLAB Function4 : MATLAB Function  TreatAsAtomicUnit=on
  MATLAB Function5 : MATLAB Function  TreatAsAtomicUnit=on
  Product{,1..5} (6 alike) : Product
  Reshape{1..6} (6 alike) : Reshape  OutputDimensionality=Column vector (2-D)
  Scope : Scope  NumInputPorts=3
  Selector{,1..5} (6 alike) : Selector  InputPortWidth=3  IndexOptions=Index vector (dialog)  Indices=1  OutputSizes=1
  Subsystem1 : Subsystem
  Subsystem2 : Subsystem
  Subsystem3 : Subsystem
  Subsystem4 : Subsystem
  Subsystem5 : Subsystem
  Subsystem6 : Subsystem
  Sum : Sum  Inputs=+|+|+
  Sum2 : Sum  Inputs=|+-
  Sum3 : Sum  Inputs=|+-
  Sum4 : Sum  Inputs=+|+
  Sum5 : Sum  Inputs=|+-
  GTQ : Outport
  wires:
  Bus Selector/1 -> Reshape1/1  "<AF_pos_G1>"
  Constant29/1 -> Product/1
  Constant28/1 -> Product/2
  Product/1 -> Gain/1
  Gain/1 -> Subsystem1/1(mg_signed)
  Subsystem1/1(COL) -> MATLAB Function/2(F)
  Reshape1/1 -> MATLAB Function/1(r)
  Bus Selector1/1 -> Reshape2/1  "<AF_pos_G2>"
  Constant6/1 -> Product3/1
  Constant5/1 -> Product3/2
  Product3/1 -> Gain3/1
  Gain3/1 -> Subsystem4/1(mg_signed)
  Subsystem4/1(COL) -> MATLAB Function1/2(F)
  Reshape2/1 -> MATLAB Function1/1(r)
  Bus Selector2/1 -> Reshape3/1  "<AF_pos_G3>"
  Constant8/1 -> Product4/1
  Constant7/1 -> Product4/2
  Product4/1 -> Gain4/1
  Gain4/1 -> Subsystem5/1(mg_signed)
  Subsystem5/1(COL) -> MATLAB Function2/2(F)
  Reshape3/1 -> MATLAB Function2/1(r)
  MATLAB Function/1(TQ) -> Selector/1
  MATLAB Function2/1(TQ) -> Selector2/1  "TQ_GRAV_at_JOINT_3"
  MATLAB Function1/1(TQ) -> Selector1/1
  Bus Creator/1 -> GTQ/1
  Selector/1 -> Sum/1
  Selector1/1 -> Sum/2
  Selector2/1 -> Sum/3  "TQ_GRAV_at_JOINT_3"
  Bus Selector3/1 -> Sum2/1  "<AF_pos_G2>"
  Constant2/1 -> Product1/1
  Constant1/1 -> Product1/2
  Product1/1 -> Gain1/1
  Gain1/1 -> Subsystem2/1(mg_signed)
  Subsystem2/1(COL) -> MATLAB Function3/2(F)
  Reshape4/1 -> MATLAB Function3/1(r)
  Bus Selector4/1 -> Sum3/1  "<AF_pos_G3>"
  Constant4/1 -> Product2/1
  Constant3/1 -> Product2/2
  Product2/1 -> Gain2/1
  Gain2/1 -> Subsystem3/1(mg_signed)
  Subsystem3/1(COL) -> MATLAB Function4/2(F)
  Reshape5/1 -> MATLAB Function4/1(r)
  Sum2/1 -> Reshape4/1
  Bus Selector3/2 -> Sum2/2  "<AF_pos_O2>"
  Bus Selector4/2 -> Sum3/2  "<AF_pos_O2>"
  Sum3/1 -> Reshape5/1
  MATLAB Function3/1(TQ) -> Selector3/1
  MATLAB Function4/1(TQ) -> Selector4/1
  Selector3/1 -> Sum4/1
  Selector4/1 -> Sum4/2
  POS/1 -> Bus Selector5/1, Bus Selector4/1, Bus Selector3/1, Bus Selector2/1, Bus Selector1/1, Bus Selector/1
  Bus Selector5/1 -> Sum5/1  "<AF_pos_G3>"
  Constant10/1 -> Product5/1
  Constant9/1 -> Product5/2
  Product5/1 -> Gain5/1
  Gain5/1 -> Subsystem6/1(mg_signed)
  Subsystem6/1(COL) -> MATLAB Function5/2(F)
  Reshape6/1 -> MATLAB Function5/1(r)
  Bus Selector5/2 -> Sum5/2  "<AF_pos_O3>"
  Sum5/1 -> Reshape6/1
  MATLAB Function5/1(TQ) -> Selector5/1
  Sum4/1 -> Scope/2, Bus Creator/2  "TQ_GRAV_at_JOINT_2"
  Sum/1 -> Scope/1, Bus Creator/1  "TQ_GRAV_at_JOINT_1"
  Selector5/1 -> Scope/3, Bus Creator/3  "TQ_GRAV_at_JOINT_3"

== system bh_4dof_LAGR_manipulator_CONTROL_DL_discrete/SIMSCAPE/Create_SM_BUS ==
  TH1 : Inport
  TH1_D : Inport  Port=2
  TH1_DD : Inport  Port=3
  TH2_DD : Inport  Port=4
  TH2_D : Inport  Port=5
  TH2 : Inport  Port=6
  TH3_DD : Inport  Port=7
  TH3_D : Inport  Port=8
  TH3 : Inport  Port=9
  TH4_DD : Inport  Port=10
  TH4_D : Inport  Port=11
  TH4 : Inport  Port=12
  Bus Creator : BusCreator  Inputs=12
  SM_BUS : Outport
  wires:
  TH2_DD/1 -> Bus Creator/4  "TH2_DD"
  TH1_DD/1 -> Bus Creator/3  "TH1_DD"
  TH1_D/1 -> Bus Creator/2  "TH1_D"
  TH2_D/1 -> Bus Creator/5  "TH2_D"
  TH1/1 -> Bus Creator/1  "TH1"
  TH2/1 -> Bus Creator/6  "TH2"
  Bus Creator/1 -> SM_BUS/1
  TH3/1 -> Bus Creator/9  "TH3"
  TH3_D/1 -> Bus Creator/8  "TH3_D"
  TH3_DD/1 -> Bus Creator/7  "TH3_DD"
  TH4/1 -> Bus Creator/12  "TH4"
  TH4_D/1 -> Bus Creator/11  "TH4_D"
  TH4_DD/1 -> Bus Creator/10  "TH4_DD"

== system bh_4dof_LAGR_manipulator_CONTROL_DL_discrete/SIMULINK_MODEL/Create_BUS ==
  TH1 : Inport
  TH1_D : Inport  Port=2
  TH1_DD : Inport  Port=3
  TH2 : Inport  Port=4
  TH2_D : Inport  Port=5
  TH2_DD : Inport  Port=6
  TH3 : Inport  Port=7
  TH3_D : Inport  Port=8
  TH3_DD : Inport  Port=9
  TH4 : Inport  Port=10
  TH4_D : Inport  Port=11
  TH4_DD : Inport  Port=12
  Bus Creator : BusCreator  Inputs=12
  SL_BUS : Outport
  wires:
  TH1_DD/1 -> Bus Creator/3  "TH1_DD"
  TH1_D/1 -> Bus Creator/2  "TH1_D"
  TH1/1 -> Bus Creator/1  "TH1"
  Bus Creator/1 -> SL_BUS/1
  TH2/1 -> Bus Creator/4  "TH2"
  TH2_D/1 -> Bus Creator/5  "TH2_D"
  TH2_DD/1 -> Bus Creator/6  "TH2_DD"
  TH3/1 -> Bus Creator/7  "TH3"
  TH3_DD/1 -> Bus Creator/9  "TH3_DD"
  TH3_D/1 -> Bus Creator/8  "TH3_D"
  TH4_DD/1 -> Bus Creator/12  "TH4_DD"
  TH4_D/1 -> Bus Creator/11  "TH4_D"
  TH4/1 -> Bus Creator/10  "TH4"

== system bh_4dof_LAGR_manipulator_CONTROL_DL_discrete/SIMULINK_MODEL/THETA_1 ==
  TH1_DD : Inport
  Constant15 : Constant  Value=theta1_0
  Constant16 : Constant  Value=theta1_dot_0
  Integrator2 : Integrator  InitialConditionSource=external
  Integrator3 : Integrator  InitialConditionSource=external
  TH1_D : Outport
  TH1 : Outport  Port=2
  wires:
  TH1_DD/1 -> Integrator2/1  "Theta1_DD"
  Constant15/1 -> Integrator3/2
  Constant16/1 -> Integrator2/2
  Integrator3/1 -> TH1/1  "Theta1"
  Integrator2/1 -> TH1_D/1, Integrator3/1  "Theta1_D"

== system bh_4dof_LAGR_manipulator_CONTROL_DL_discrete/SIMULINK_MODEL/THETA_2 ==
  TH2_DD : Inport
  Constant15 : Constant  Value=theta2_0
  Constant16 : Constant  Value=theta2_dot_0
  Integrator2 : Integrator  InitialConditionSource=external
  Integrator3 : Integrator  InitialConditionSource=external
  TH2_D : Outport
  TH2 : Outport  Port=2
  wires:
  TH2_DD/1 -> Integrator2/1  "Theta2_DD"
  Integrator2/1 -> TH2_D/1, Integrator3/1  "Theta2_D"
  Constant15/1 -> Integrator3/2
  Constant16/1 -> Integrator2/2
  Integrator3/1 -> TH2/1  "Theta2"

== system bh_4dof_LAGR_manipulator_CONTROL_DL_discrete/SIMULINK_MODEL/THETA_3 ==
  TH3_DD : Inport
  Constant15 : Constant  Value=theta3_0
  Constant16 : Constant  Value=theta3_dot_0
  Integrator2 : Integrator  InitialConditionSource=external
  Integrator3 : Integrator  InitialConditionSource=external
  TH3_D : Outport
  TH3 : Outport  Port=2
  wires:
  TH3_DD/1 -> Integrator2/1  "Theta3_DD"
  Integrator2/1 -> TH3_D/1, Integrator3/1  "Theta3_D"
  Constant15/1 -> Integrator3/2
  Constant16/1 -> Integrator2/2
  Integrator3/1 -> TH3/1  "Theta3"

== system bh_4dof_LAGR_manipulator_CONTROL_DL_discrete/SIMULINK_MODEL/THETA_4 ==
  TH4_DD : Inport
  Constant15 : Constant  Value=theta4_0
  Constant16 : Constant  Value=theta4_dot_0
  Integrator2 : Integrator  InitialConditionSource=external
  Integrator3 : Integrator  InitialConditionSource=external
  TH4_D : Outport
  TH4 : Outport  Port=2
  wires:
  TH4_DD/1 -> Integrator2/1  "Theta4_DD"
  Integrator2/1 -> TH4_D/1, Integrator3/1  "Theta4_D"
  Constant15/1 -> Integrator3/2
  Constant16/1 -> Integrator2/2
  Integrator3/1 -> TH4/1  "Theta4"

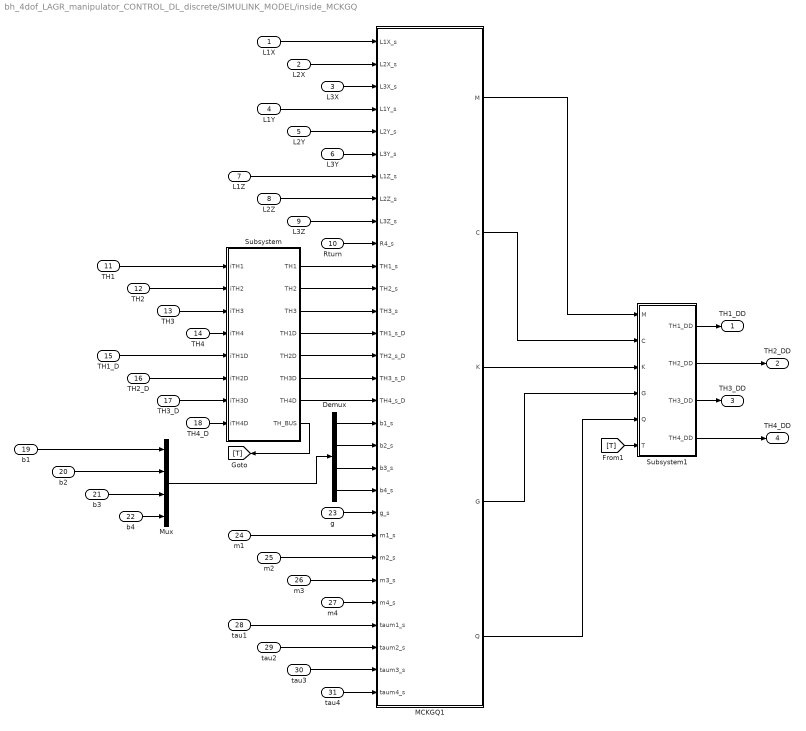
== system bh_4dof_LAGR_manipulator_CONTROL_DL_discrete/SIMULINK_MODEL/inside_MCKGQ ==
  L1X : Inport
  L2X : Inport  Port=2
  L3X : Inport  Port=3
  L1Y : Inport  Port=4
  L2Y : Inport  Port=5
  L3Y : Inport  Port=6
  L1Z : Inport  Port=7
  L2Z : Inport  Port=8
  L3Z : Inport  Port=9
  Rturn : Inport  Port=10
  TH1 : Inport  Port=11
  TH2 : Inport  Port=12
  TH3 : Inport  Port=13
  TH4 : Inport  Port=14
  TH1_D : Inport  Port=15
  TH2_D : Inport  Port=16
  TH3_D : Inport  Port=17
  TH4_D : Inport  Port=18
  b1 : Inport  Port=19
  b2 : Inport  Port=20
  b3 : Inport  Port=21
  b4 : Inport  Port=22
  g : Inport  Port=23
  m1 : Inport  Port=24
  m2 : Inport  Port=25
  m3 : Inport  Port=26
  m4 : Inport  Port=27
  tau1 : Inport  Port=28
  tau2 : Inport  Port=29
  tau3 : Inport  Port=30
  tau4 : Inport  Port=31
  Demux : Demux
  MCKGQ1 : MATLAB Function  TreatAsAtomicUnit=on
  Mux : Mux
  Subsystem : Subsystem
  Subsystem1 : Subsystem
  TH1_DD : Outport
  TH2_DD : Outport  Port=2
  TH3_DD : Outport  Port=3
  TH4_DD : Outport  Port=4
  wires:
  m2/1 -> MCKGQ1/24(m2_s)
  m3/1 -> MCKGQ1/25(m3_s)
  m4/1 -> MCKGQ1/26(m4_s)
  tau1/1 -> MCKGQ1/27(taum1_s)
  g/1 -> MCKGQ1/22(g_s)
  m1/1 -> MCKGQ1/23(m1_s)
  TH1_D/1 -> Subsystem/5(iTH1D)
  b1/1 -> Mux/1
  b2/1 -> Mux/2
  TH3/1 -> Subsystem/3(iTH3)
  b3/1 -> Mux/3
  TH4_D/1 -> Subsystem/8(iTH4D)
  TH2_D/1 -> Subsystem/6(iTH2D)
  TH3_D/1 -> Subsystem/7(iTH3D)
  b4/1 -> Mux/4
  tau2/1 -> MCKGQ1/28(taum2_s)
  tau3/1 -> MCKGQ1/29(taum3_s)
  tau4/1 -> MCKGQ1/30(taum4_s)
  L2X/1 -> MCKGQ1/2(L2X_s)
  L3X/1 -> MCKGQ1/3(L3X_s)
  L2Y/1 -> MCKGQ1/5(L2Y_s)
  L3Y/1 -> MCKGQ1/6(L3Y_s)
  L1Y/1 -> MCKGQ1/4(L1Y_s)
  L2Z/1 -> MCKGQ1/8(L2Z_s)
  L3Z/1 -> MCKGQ1/9(L3Z_s)
  L1Z/1 -> MCKGQ1/7(L1Z_s)
  TH1/1 -> Subsystem/1(iTH1)
  Rturn/1 -> MCKGQ1/10(R4_s)
  TH2/1 -> Subsystem/2(iTH2)
  L1X/1 -> MCKGQ1/1(L1X_s)
  Subsystem/8(TH_BUS) -> [T]
  Subsystem/7(TH4D) -> MCKGQ1/17(TH4_s_D)
  Subsystem/6(TH3D) -> MCKGQ1/16(TH3_s_D)
  Subsystem/5(TH2D) -> MCKGQ1/15(TH2_s_D)
  Subsystem/4(TH1D) -> MCKGQ1/14(TH1_s_D)
  Subsystem/3(TH3) -> MCKGQ1/13(TH3_s)
  Subsystem/2(TH2) -> MCKGQ1/12(TH2_s)
  Subsystem/1(TH1) -> MCKGQ1/11(TH1_s)
  TH4/1 -> Subsystem/4(iTH4)
  Demux/1 -> MCKGQ1/18(b1_s)
  Demux/2 -> MCKGQ1/19(b2_s)
  Demux/3 -> MCKGQ1/20(b3_s)
  Demux/4 -> MCKGQ1/21(b4_s)
  Mux/1 -> Demux/1
  Subsystem1/1(TH1_DD) -> TH1_DD/1
  Subsystem1/2(TH2_DD) -> TH2_DD/1
  MCKGQ1/1(M) -> Subsystem1/1(M)
  MCKGQ1/2(C) -> Subsystem1/2(C)
  MCKGQ1/3(K) -> Subsystem1/3(K)
  MCKGQ1/4(G) -> Subsystem1/4(G)
  MCKGQ1/5(Q) -> Subsystem1/5(Q)
  [T] -> Subsystem1/6(T)
  Subsystem1/3(TH3_DD) -> TH3_DD/1
  Subsystem1/4(TH4_DD) -> TH4_DD/1

== system bh_4dof_LAGR_manipulator_CONTROL_DL_discrete/TRAJECTORY/End_Eff_Traj ==
  Bus Creator : BusCreator  Inputs=8
  Demux : Demux  Outputs=3
  Demux1 : Demux  Outputs=3
  From Spreadsheet : FromSpreadsheet  FileName=bh_hello_complete.xlsx  SheetName=COMP_SPLINE _4dof  SampleTime=0.01  ExtrapolationBeforeFirstDataPoint=Hold first value  ExtrapolationAfterLastDataPoint=Hold last value
  Mux : Mux  Inputs=3
  Mux1 : Mux  Inputs=3
  Reshape : Reshape  OutputDimensionality=Column vector (2-D)
  Reshape1 : Reshape  OutputDimensionality=Column vector (2-D)
  EFF_TRAJ : Outport
  wires:
  From Spreadsheet/2 -> Mux/2  "YE"
  From Spreadsheet/3 -> Mux/3  "ZE"
  From Spreadsheet/1 -> Mux/1  "XE"
  From Spreadsheet/4 -> Mux1/1  "DXEDT"
  Bus Creator/1 -> EFF_TRAJ/1
  From Spreadsheet/6 -> Mux1/3  "DZEDT"
  From Spreadsheet/5 -> Mux1/2  "DYEDT"
  Demux/1 -> Bus Creator/6  "DXEDT"
  Demux/2 -> Bus Creator/7  "DYEDT"
  Demux/3 -> Bus Creator/8  "DZEDT"
  Demux1/1 -> Bus Creator/1  "XE"
  Demux1/2 -> Bus Creator/2  "YE"
  Demux1/3 -> Bus Creator/3  "ZE"
  Mux/1 -> Reshape/1  "XYZ"
  Mux1/1 -> Reshape1/1
  Reshape/1 -> Bus Creator/4, Demux1/1  "XYZ_POS"
  Reshape1/1 -> Demux/1, Bus Creator/5  "XYZ_VEL"

== system bh_4dof_LAGR_manipulator_CONTROL_DL_discrete/TRAJECTORY/Subsystem ==
  In1 : Inport
  In2 : Inport  Port=2
  Mux2 : Mux  Inputs=2
  Reshape : Reshape  OutputDimensionality=Column vector (2-D)
  Reshape1 : Reshape  OutputDimensionality=Column vector (2-D)
  Selector : Selector  InputPortWidth=8  IndexOptions=Index vector (dialog)  Indices=[1 5]  OutputSizes=1
  Selector1 : Selector  InputPortWidth=8  IndexOptions=Index vector (dialog)  Indices=[2 6]  OutputSizes=1
  Selector2 : Selector  InputPortWidth=8  IndexOptions=Index vector (dialog)  Indices=[3 7]  OutputSizes=1
  Selector3 : Selector  InputPortWidth=8  IndexOptions=Index vector (dialog)  Indices=[4 8]  OutputSizes=1
  Out1 : Outport
  Out2 : Outport  Port=2
  Out3 : Outport  Port=3
  Out4 : Outport  Port=4
  wires:
  In1/1 -> Reshape/1
  In2/1 -> Reshape1/1
  Reshape/1 -> Mux2/1
  Reshape1/1 -> Mux2/2
  Selector2/1 -> Out3/1
  Selector1/1 -> Out2/1
  Selector/1 -> Out1/1
  Mux2/1 -> Selector1/1, Selector/1, Selector2/1, Selector3/1
  Selector3/1 -> Out4/1

== system bh_4dof_LAGR_manipulator_CONTROL_DL_discrete/TRAJECTORY/XY_compare ==
  XY_GOAL : Inport
  XY : Inport  Port=2
  Bus Selector1 : BusSelector  OutputSignals=XE,YE,ZE
  Demux : Demux  Outputs=3
  Mux : Mux  Inputs=2
  Mux1 : Mux  Inputs=2
  Mux2 : Mux  Inputs=2
  X : Outport
  Y : Outport  Port=2
  Z : Outport  Port=3
  wires:
  XY_GOAL/1 -> Bus Selector1/1
  XY/1 -> Demux/1
  Bus Selector1/1 -> Mux/1  "<XE>"
  Demux/1 -> Mux/2
  Bus Selector1/2 -> Mux1/1  "<YE>"
  Demux/2 -> Mux1/2
  Mux/1 -> X/1
  Mux1/1 -> Y/1
  Mux2/1 -> Z/1
  Bus Selector1/3 -> Mux2/1  "<ZE>"
  Demux/3 -> Mux2/2

== system bh_4dof_LAGR_manipulator_CONTROL_DL_discrete/TRAJECTORY/get_XYDOT ==
  In1 : Inport
  Bus Selector2 : BusSelector  OutputSignals=DXEDT,DYEDT,DZEDT
  Mux2 : Mux  Inputs=3
  Reshape : Reshape  OutputDimensionality=Column vector (2-D)
  Out1 : Outport
  wires:
  Bus Selector2/1 -> Mux2/1  "<DXEDT>"
  Bus Selector2/2 -> Mux2/2  "<DYEDT>"
  In1/1 -> Bus Selector2/1
  Mux2/1 -> Reshape/1
  Reshape/1 -> Out1/1  "XY_DOT"
  Bus Selector2/3 -> Mux2/3  "<DZEDT>"

== system bh_4dof_LAGR_manipulator_CONTROL_DL_discrete/VIEW/XYZ_EFF_COMPARE ==
  CMD_BUS : Inport
  PLANT_BUS : Inport  Port=2
  Bus Selector1 : BusSelector  OutputSignals=CALC_POS_BUS.WF_pos_EFF
  Bus Selector4 : BusSelector  OutputSignals=XYZ_BUS.XYZ_POS
  Mux : Mux  Inputs=2
  Reshape1 : Reshape  OutputDimensionality=Column vector (2-D)
  Reshape2 : Reshape  OutputDimensionality=Column vector (2-D)
  Selector : Selector  InputPortWidth=6  IndexOptions=Index vector (dialog)  Indices=[1 4]  OutputSizes=1
  Selector1 : Selector  InputPortWidth=6  IndexOptions=Index vector (dialog)  Indices=[2 5]  OutputSizes=1
  Selector2 : Selector  InputPortWidth=6  IndexOptions=Index vector (dialog)  Indices=[3 6]  OutputSizes=1
  X : Outport
  Y : Outport  Port=2
  Z : Outport  Port=3
  wires:
  CMD_BUS/1 -> Bus Selector4/1
  PLANT_BUS/1 -> Bus Selector1/1
  Bus Selector4/1 -> Reshape1/1  "<XYZ_POS>"
  Bus Selector1/1 -> Reshape2/1  "<WF_pos_EFF>"
  Reshape1/1 -> Mux/1
  Reshape2/1 -> Mux/2
  Mux/1 -> Selector2/1, Selector1/1, Selector/1
  Selector2/1 -> Z/1
  Selector1/1 -> Y/1
  Selector/1 -> X/1

== system bh_4dof_LAGR_manipulator_CONTROL_DL_discrete/Create_PLANT_BUS/Subsystem1/Subsystem1 ==
  mg_signed : Inport
  Constant : Constant  Value=0
  Mux : Mux  Inputs=3
  Reshape : Reshape  OutputDimensionality=Column vector (2-D)
  COL : Outport
  wires:
  mg_signed/1 -> Mux/3
  Constant/1 -> Mux/2, Mux/1
  Mux/1 -> Reshape/1
  Reshape/1 -> COL/1

== system bh_4dof_LAGR_manipulator_CONTROL_DL_discrete/Create_PLANT_BUS/Subsystem1/Subsystem2 ==
  mg_signed : Inport
  Constant : Constant  Value=0
  Mux : Mux  Inputs=3
  Reshape : Reshape  OutputDimensionality=Column vector (2-D)
  COL : Outport
  wires:
  mg_signed/1 -> Mux/3
  Constant/1 -> Mux/2, Mux/1
  Mux/1 -> Reshape/1
  Reshape/1 -> COL/1

== system bh_4dof_LAGR_manipulator_CONTROL_DL_discrete/Create_PLANT_BUS/Subsystem1/Subsystem3 ==
  mg_signed : Inport
  Constant : Constant  Value=0
  Mux : Mux  Inputs=3
  Reshape : Reshape  OutputDimensionality=Column vector (2-D)
  COL : Outport
  wires:
  mg_signed/1 -> Mux/3
  Constant/1 -> Mux/2, Mux/1
  Mux/1 -> Reshape/1
  Reshape/1 -> COL/1

== system bh_4dof_LAGR_manipulator_CONTROL_DL_discrete/Create_PLANT_BUS/Subsystem1/Subsystem4 ==
  mg_signed : Inport
  Constant : Constant  Value=0
  Mux : Mux  Inputs=3
  Reshape : Reshape  OutputDimensionality=Column vector (2-D)
  COL : Outport
  wires:
  mg_signed/1 -> Mux/3
  Constant/1 -> Mux/2, Mux/1
  Mux/1 -> Reshape/1
  Reshape/1 -> COL/1

== system bh_4dof_LAGR_manipulator_CONTROL_DL_discrete/Create_PLANT_BUS/Subsystem1/Subsystem5 ==
  mg_signed : Inport
  Constant : Constant  Value=0
  Mux : Mux  Inputs=3
  Reshape : Reshape  OutputDimensionality=Column vector (2-D)
  COL : Outport
  wires:
  mg_signed/1 -> Mux/3
  Constant/1 -> Mux/2, Mux/1
  Mux/1 -> Reshape/1
  Reshape/1 -> COL/1

== system bh_4dof_LAGR_manipulator_CONTROL_DL_discrete/Create_PLANT_BUS/Subsystem1/Subsystem6 ==
  mg_signed : Inport
  Constant : Constant  Value=0
  Mux : Mux  Inputs=3
  Reshape : Reshape  OutputDimensionality=Column vector (2-D)
  COL : Outport
  wires:
  mg_signed/1 -> Mux/3
  Constant/1 -> Mux/2, Mux/1
  Mux/1 -> Reshape/1
  Reshape/1 -> COL/1

== system bh_4dof_LAGR_manipulator_CONTROL_DL_discrete/Create_PLANT_BUS1/Subsystem1/Subsystem1 ==
  mg_signed : Inport
  Constant : Constant  Value=0
  Mux : Mux  Inputs=3
  Reshape : Reshape  OutputDimensionality=Column vector (2-D)
  COL : Outport
  wires:
  mg_signed/1 -> Mux/3
  Constant/1 -> Mux/2, Mux/1
  Mux/1 -> Reshape/1
  Reshape/1 -> COL/1

== system bh_4dof_LAGR_manipulator_CONTROL_DL_discrete/Create_PLANT_BUS1/Subsystem1/Subsystem2 ==
  mg_signed : Inport
  Constant : Constant  Value=0
  Mux : Mux  Inputs=3
  Reshape : Reshape  OutputDimensionality=Column vector (2-D)
  COL : Outport
  wires:
  mg_signed/1 -> Mux/3
  Constant/1 -> Mux/2, Mux/1
  Mux/1 -> Reshape/1
  Reshape/1 -> COL/1

== system bh_4dof_LAGR_manipulator_CONTROL_DL_discrete/Create_PLANT_BUS1/Subsystem1/Subsystem3 ==
  mg_signed : Inport
  Constant : Constant  Value=0
  Mux : Mux  Inputs=3
  Reshape : Reshape  OutputDimensionality=Column vector (2-D)
  COL : Outport
  wires:
  mg_signed/1 -> Mux/3
  Constant/1 -> Mux/2, Mux/1
  Mux/1 -> Reshape/1
  Reshape/1 -> COL/1

== system bh_4dof_LAGR_manipulator_CONTROL_DL_discrete/Create_PLANT_BUS1/Subsystem1/Subsystem4 ==
  mg_signed : Inport
  Constant : Constant  Value=0
  Mux : Mux  Inputs=3
  Reshape : Reshape  OutputDimensionality=Column vector (2-D)
  COL : Outport
  wires:
  mg_signed/1 -> Mux/3
  Constant/1 -> Mux/2, Mux/1
  Mux/1 -> Reshape/1
  Reshape/1 -> COL/1

== system bh_4dof_LAGR_manipulator_CONTROL_DL_discrete/Create_PLANT_BUS1/Subsystem1/Subsystem5 ==
  mg_signed : Inport
  Constant : Constant  Value=0
  Mux : Mux  Inputs=3
  Reshape : Reshape  OutputDimensionality=Column vector (2-D)
  COL : Outport
  wires:
  mg_signed/1 -> Mux/3
  Constant/1 -> Mux/2, Mux/1
  Mux/1 -> Reshape/1
  Reshape/1 -> COL/1

== system bh_4dof_LAGR_manipulator_CONTROL_DL_discrete/Create_PLANT_BUS1/Subsystem1/Subsystem6 ==
  mg_signed : Inport
  Constant : Constant  Value=0
  Mux : Mux  Inputs=3
  Reshape : Reshape  OutputDimensionality=Column vector (2-D)
  COL : Outport
  wires:
  mg_signed/1 -> Mux/3
  Constant/1 -> Mux/2, Mux/1
  Mux/1 -> Reshape/1
  Reshape/1 -> COL/1
